simulink model "SprayDryer_with_Heater_FOPDT"  (R2018a)
settings: Solver=VariableStepAuto  StartTime=0.0  StopTime=60  FixedStep=0.01  RelTol=1e-3
values from neighbouring files (symbols this model uses):
  finalSetpoint = 1    [SprayDryer_FOPDT_CaseStudy1.m]    (also in SprayDryer_FOPDT_CaseStudy2.m; SprayDryer_with_Heater_FOPDT_CaseStudy1.m)
  initialSetpoint = 0    [SprayDryer_FOPDT_CaseStudy1.m]    (also in SprayDryer_FOPDT_CaseStudy2.m; SprayDryer_with_Heater_FOPDT_CaseStudy1.m)
  K_heater = 5.8    [SprayDryer_with_Heater_FOPDT_CaseStudy1.m]
  K_process = 2    [SprayDryer_FOPDT_CaseStudy1.m]    (also in SprayDryer_FOPDT_CaseStudy2.m = 0.86; SprayDryer_with_Heater_FOPDT_CaseStudy1.m)
  kD_controller = kP_controller*tauD_controller    (= 0)    [SprayDryer_FOPDT_CaseStudy1.m]    (also in SprayDryer_FOPDT_CaseStudy2.m; SprayDryer_with_Heater_FOPDT_CaseStudy1.m)
  kI_controller = kP_controller/tauI_controller    (= 0.504860221536)    [SprayDryer_FOPDT_CaseStudy1.m]    (also in SprayDryer_FOPDT_CaseStudy2.m; SprayDryer_with_Heater_FOPDT_CaseStudy1.m = 2)
  kP_controller = 2.68    [SprayDryer_FOPDT_CaseStudy1.m]    (also in SprayDryer_FOPDT_CaseStudy2.m; SprayDryer_with_Heater_FOPDT_CaseStudy1.m = 0.01)
  tau_heater = 1    [SprayDryer_with_Heater_FOPDT_CaseStudy1.m]
  tau_process = 6.8    [SprayDryer_FOPDT_CaseStudy1.m]    (also in SprayDryer_FOPDT_CaseStudy2.m = 2.44; SprayDryer_with_Heater_FOPDT_CaseStudy1.m)
  theta_heater = 7.3/60    (= 0.121666666667)    [SprayDryer_with_Heater_FOPDT_CaseStudy1.m]
  theta_process = 1    [SprayDryer_FOPDT_CaseStudy1.m]    (also in SprayDryer_FOPDT_CaseStudy2.m = 0.16; SprayDryer_with_Heater_FOPDT_CaseStudy1.m)
  timeSetpointChange = 10    [SprayDryer_FOPDT_CaseStudy1.m]    (also in SprayDryer_FOPDT_CaseStudy2.m; SprayDryer_with_Heater_FOPDT_CaseStudy1.m)
libraries: simulink x1
settings Model: Creator=sadbo  LastModifiedBy=sadbo
settings DataIOCC: SaveFormat=Structure  SaveOutput=off  DSMLogging=off

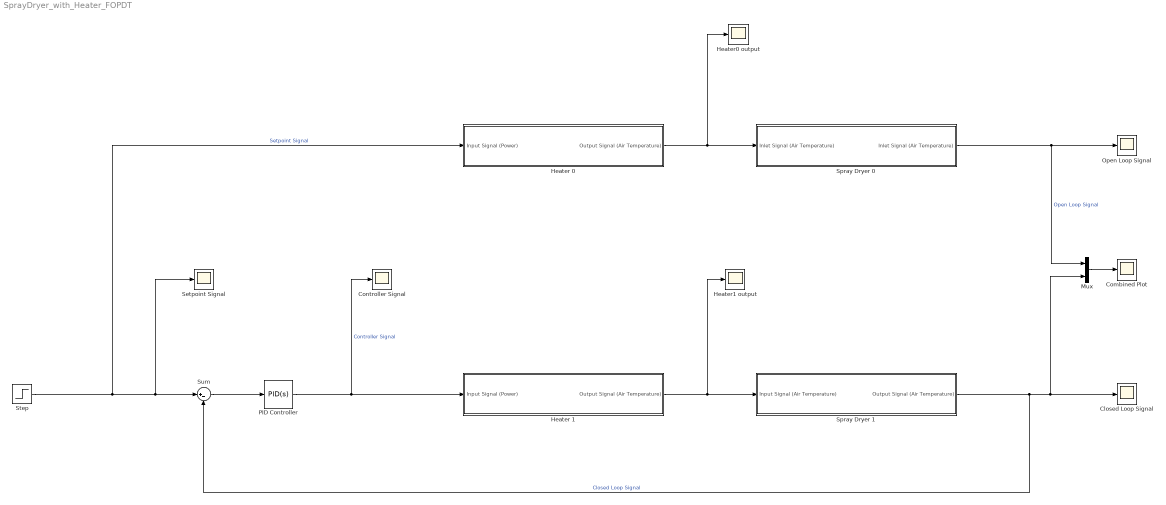
== system SprayDryer_with_Heater_FOPDT ==
  "Closed Loop Signal " : Scope
  "Combined Plot " : Scope
  Controller Signal : Scope
  "Heater 0 " : Subsystem
  "Heater 1 " : Subsystem
  Heater0 output : Scope
  Heater1 output : Scope
  Mux : Mux  Inputs=2
  "Open Loop Signal " : Scope
  PID Controller : simulink/Continuous/PID Controller  Controller=PID  TimeDomain=Continuous-time  SampleTime=-1  IntegratorMethod=Forward Euler  FilterMethod=Forward Euler  Form=Ideal  UseFilter=on  ControllerParametersSource=internal  P=kP_controller  I=kI_controller  D=kD_controller  N=0  InitialConditionSource=internal  InitialConditionForIntegrator=0  InitialConditionForFilter=0  ExternalReset=none  LimitOutput=off  UpperSaturationLimit=inf  LowerSaturationLimit=-inf  LinearizeAsGain=on  AntiWindupMode=none  Kb=1  TrackingMode=off  Kt=1  PParamMin=[]  PParamMax=[]  IParamMin=[]  IParamMax=[]  DParamMin=[]  DParamMax=[]  NParamMin=[]  NParamMax=[]  KbParamMin=[]  KbParamMax=[]  KtParamMin=[]  KtParamMax=[]  POutMin=[]  POutMax=[]  IOutMin=[]  IOutMax=[]  DOutMin=[]  DOutMax=[]  NOutMin=[]  NOutMax=[]  KbOutMin=[]  KbOutMax=[]  KtOutMin=[]  KtOutMax=[]  IntegratorOutMin=[]  IntegratorOutMax=[]  FilterOutMin=[]  FilterOutMax=[]  SumOutMin=[]  SumOutMax=[]  SumI1OutMin=[]  SumI1OutMax=[]  SumI2OutMin=[]  SumI2OutMax=[]  SumI3OutMin=[]  SumI3OutMax=[]  SumDOutMin=[]  SumDOutMax=[]  SaturationOutMin=[]  SaturationOutMax=[]  IntegratorContinuousStateAttributes=''  IntegratorStateMustResolveToSignalObject=off  IntegratorRTWStateStorageClass=Auto  FilterContinuousStateAttributes=''  FilterStateMustResolveToSignalObject=off  FilterRTWStateStorageClass=Auto  DifferentiatorICPrevScaledInput=0  DifferentiatorOutMin=[]  DifferentiatorOutMax=[]  FilterDiffOutCoefMin=[]  FilterDiffOutCoefMax=[]  SumDenOutMin=[]  SumDenOutMax=[]  SumNumOutMin=[]  SumNumOutMax=[]  ReciprocalOutMin=[]  ReciprocalOutMax=[]  DivideOutMin=[]  DivideOutMax=[]  TunerSelectOption=Transfer Function Based (PID Tuner App)
  Setpoint Signal : Scope
  "Spray Dryer 0 " : Subsystem
  Spray Dryer 1 : Subsystem
  "Step " : Step  Time=timeSetpointChange  Before=initialSetpoint  After=finalSetpoint  SampleTime=0
  Sum : Sum  Inputs=|+-
  wires:
  Sum/1 -> PID Controller/1
  Spray Dryer 1/1("Output Signal (Air Temperature) ") -> Mux/2, "Closed Loop Signal "/1, Sum/2  "Closed Loop Signal"
  PID Controller/1 -> "Heater 1 "/1(Input Signal (Power)), Controller Signal/1  "Controller Signal"
  "Spray Dryer 0 "/1("Inlet Signal (Air Temperature) ") -> Mux/1, "Open Loop Signal "/1  "Open Loop Signal"
  Mux/1 -> "Combined Plot "/1
  "Step "/1 -> "Heater 0 "/1(Input Signal (Power)), Setpoint Signal/1, Sum/1  "Setpoint Signal"
  "Heater 1 "/1("Output Signal (Air Temperature) ") -> Heater1 output/1, Spray Dryer 1/1(Input Signal (Air Temperature))
  "Heater 0 "/1("Output Signal (Air Temperature) ") -> Heater0 output/1, "Spray Dryer 0 "/1(Inlet Signal (Air Temperature))

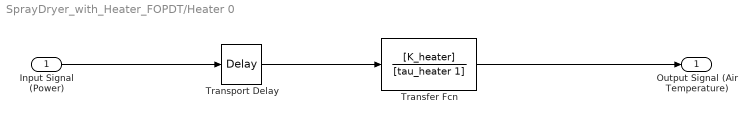
== system SprayDryer_with_Heater_FOPDT/Heater 0  ==
  Input Signal (Power) : Inport
  Transfer Fcn : TransferFcn  Numerator=[K_heater]  Denominator=[tau_heater 1]
  Transport Delay : TransportDelay  DelayTime=theta_heater
  "Output Signal (Air Temperature) " : Outport
  wires:
  Transport Delay/1 -> Transfer Fcn/1
  Transfer Fcn/1 -> "Output Signal (Air Temperature) "/1
  Input Signal (Power)/1 -> Transport Delay/1

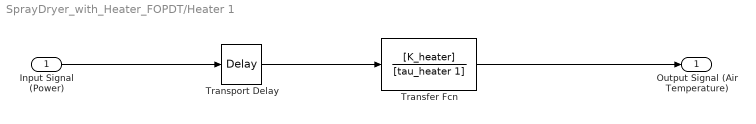
== system SprayDryer_with_Heater_FOPDT/Heater 1  ==
  Input Signal (Power) : Inport
  Transfer Fcn : TransferFcn  Numerator=[K_heater]  Denominator=[tau_heater 1]
  Transport Delay : TransportDelay  DelayTime=theta_heater
  "Output Signal (Air Temperature) " : Outport
  wires:
  Transport Delay/1 -> Transfer Fcn/1
  Transfer Fcn/1 -> "Output Signal (Air Temperature) "/1
  Input Signal (Power)/1 -> Transport Delay/1

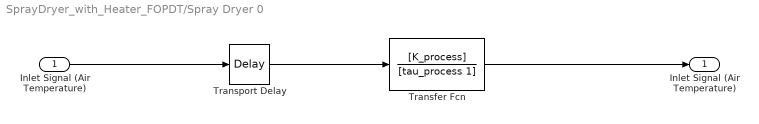
== system SprayDryer_with_Heater_FOPDT/Spray Dryer 0  ==
  Inlet Signal (Air Temperature) : Inport
  Transfer Fcn : TransferFcn  Numerator=[K_process]  Denominator=[tau_process 1]
  Transport Delay : TransportDelay  DelayTime=theta_process
  "Inlet Signal (Air Temperature) " : Outport
  wires:
  Inlet Signal (Air Temperature)/1 -> Transport Delay/1
  Transfer Fcn/1 -> "Inlet Signal (Air Temperature) "/1
  Transport Delay/1 -> Transfer Fcn/1

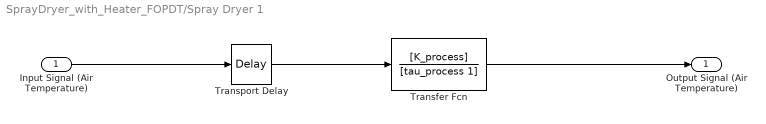
== system SprayDryer_with_Heater_FOPDT/Spray Dryer 1 ==
  Input Signal (Air Temperature) : Inport
  Transfer Fcn : TransferFcn  Numerator=[K_process]  Denominator=[tau_process 1]
  Transport Delay : TransportDelay  DelayTime=theta_process
  "Output Signal (Air Temperature) " : Outport
  wires:
  Input Signal (Air Temperature)/1 -> Transport Delay/1
  Transfer Fcn/1 -> "Output Signal (Air Temperature) "/1
  Transport Delay/1 -> Transfer Fcn/1
